simulink model "Fusion_Frame_Model_Architecture"  (R2018a)
settings: Solver=FixedStepAuto  StartTime=0.0  StopTime=SimulationTime  FixedStep=SamplingTime  RelTol=1e-3
undefined symbols (not defined in the file or in its folder): ACTIVATE_CAM, ACTIVATE_RAD, CAM1_detTimeStamp, CAM1_MeasNoise, CAM1_objClassID, CAM1_PX, CAM1_PY, CAM1_VX, CAM1_VY, CAM2_detTimeStamp, CAM2_MeasNoise, CAM2_objClassID, CAM2_PX, CAM2_PY, CAM2_VX, CAM2_VY, CAM3_detTimeStamp, CAM3_MeasNoise, CAM3_objClassID, CAM3_PX, CAM3_PY, CAM3_VX, CAM3_VY, CAM4_detTimeStamp, CAM4_MeasNoise, CAM4_objClassID, CAM4_PX, CAM4_PY, CAM4_VX, CAM4_VY, CAM5_detTimeStamp, CAM5_MeasNoise, CAM5_objClassID, CAM5_PX, CAM5_PY, CAM5_VX, CAM5_VY, CAM6_detTimeStamp, CAM6_MeasNoise, CAM6_objClassID, CAM6_PX, CAM6_PY, CAM6_VX, CAM6_VY, CAM7_detTimeStamp, CAM7_MeasNoise, CAM7_objClassID, CAM7_PX, CAM7_PY, CAM7_VX, CAM7_VY, CAM8_detTimeStamp, CAM8_MeasNoise, CAM8_objClassID, CAM8_PX, CAM8_PY, CAM8_VX, CAM8_VY, CAM_nMeas, CAM_TYPE ... (+181)
libraries: simulink_extras x4
(part 8 of 11)

== system Fusion_Frame_Model_Architecture/SENSOR_FUSION_SYSTEM/OBJECT_TRACKER_SENSOR_FUSION/SENSOR_LAYOUT_AND_CHRACTERIZATION/PRE_COMPUTE_SENSOR_FOV_GRID/CREATE_GRID/For Iterator Subsystem ==
  xIndex : Inport
  Cy : Inport  Port=2
  GridParam : Inport  Port=3
  CellIDArray : Inport  Port=4
  Compute_Grid_Cell_Cartesian_Coordinate : Subsystem
  Compute_Grid_Cell_Discreete_Index : Subsystem
  For Iterator : ForIterator  ResetStates=reset  IterationSource=external
  SET_DATA : Subsystem
  Terminator : Terminator
  Terminator1 : Terminator
  CellIDVectorUpd : Outport
  wires:
  Cy/1 -> For Iterator/1
  xIndex/1 -> Compute_Grid_Cell_Cartesian_Coordinate/2(x_Index)
  GridParam/1 -> Compute_Grid_Cell_Cartesian_Coordinate/1(GridParam), Compute_Grid_Cell_Discreete_Index/1(GridParam)
  Compute_Grid_Cell_Cartesian_Coordinate/2(y_Coordinate) -> Compute_Grid_Cell_Discreete_Index/3(y_coord)
  Compute_Grid_Cell_Cartesian_Coordinate/1(x_Coordinate) -> Compute_Grid_Cell_Discreete_Index/2(x_coord)
  For Iterator/1 -> Compute_Grid_Cell_Cartesian_Coordinate/3(y_Index)
  CellIDArray/1 -> SET_DATA/1(CellIDArray)
  SET_DATA/1(CellIDArrayUpd) -> CellIDVectorUpd/1
  Compute_Grid_Cell_Discreete_Index/1(CellID_x) -> Terminator/1
  Compute_Grid_Cell_Discreete_Index/2(CellID_y) -> Terminator1/1
  Compute_Grid_Cell_Discreete_Index/3(CellID) -> SET_DATA/2(CellID)

== system Fusion_Frame_Model_Architecture/SENSOR_FUSION_SYSTEM/OBJECT_TRACKER_SENSOR_FUSION/SENSOR_LAYOUT_AND_CHRACTERIZATION/SET_SENSOR_CALLIBRATION_PARAMETER/SET_CAMERA_SENSOR_PARAM/GET_DATA ==
  CAMSnsrParam : Inport
  Bus Selector : BusSelector  OutputSignals=CameraIntrinsics,CameraExtrinsics
  CameraIntrinsics : Outport
  CameraExtrinsics : Outport  Port=2
  wires:
  CAMSnsrParam/1 -> Bus Selector/1
  Bus Selector/2 -> CameraExtrinsics/1  "<CameraExtrinsics>"
  Bus Selector/1 -> CameraIntrinsics/1  "<CameraIntrinsics>"

== system Fusion_Frame_Model_Architecture/SENSOR_FUSION_SYSTEM/OBJECT_TRACKER_SENSOR_FUSION/SENSOR_LAYOUT_AND_CHRACTERIZATION/SET_SENSOR_CALLIBRATION_PARAMETER/SET_CAMERA_SENSOR_PARAM/SET_CAMERA_EXTRINSIC_PARAM ==
  CameraCalibParam : Inport
  INSTALLED_CAMERA_i : ForIterator  IterationLimit=nCameras
  SET_CAMERA_EXTRINSIC_PARAM : Subsystem
  CameraCalibParamSet : Outport
  wires:
  INSTALLED_CAMERA_i/1 -> SET_CAMERA_EXTRINSIC_PARAM/2(SensorID)
  SET_CAMERA_EXTRINSIC_PARAM/1(Out1) -> CameraCalibParamSet/1
  CameraCalibParam/1 -> SET_CAMERA_EXTRINSIC_PARAM/1(SensorParam)

== system Fusion_Frame_Model_Architecture/SENSOR_FUSION_SYSTEM/OBJECT_TRACKER_SENSOR_FUSION/SENSOR_LAYOUT_AND_CHRACTERIZATION/SET_SENSOR_CALLIBRATION_PARAMETER/SET_CAMERA_SENSOR_PARAM/SET_CAMERA_INTRINSIC_PARAM ==
  CameraCalibParam : Inport
  CAMERA_TYPE_i : ForIterator  IterationLimit=nCameraTypes
  SET_CAMERA_INTRINSIC_PARAM : Subsystem
  CameraCalibParamSet : Outport
  wires:
  CameraCalibParam/1 -> SET_CAMERA_INTRINSIC_PARAM/1(SensorParam)
  CAMERA_TYPE_i/1 -> SET_CAMERA_INTRINSIC_PARAM/2(SensorID)
  SET_CAMERA_INTRINSIC_PARAM/1(Out1) -> CameraCalibParamSet/1

== system Fusion_Frame_Model_Architecture/SENSOR_FUSION_SYSTEM/OBJECT_TRACKER_SENSOR_FUSION/SENSOR_LAYOUT_AND_CHRACTERIZATION/SET_SENSOR_CALLIBRATION_PARAMETER/SET_CAMERA_SENSOR_PARAM/SET_DATA ==
  CameraIntrinsics : Inport
  CameraExtrinsics : Inport  Port=2
  Bus Creator : BusCreator  Inputs=2  OutDataTypeStr=Bus: CAM_SENSOR_PARAM  NonVirtualBus=on
      settings: InheritFromInputs=off
  CAMSnsrParamUpd : Outport
  wires:
  Bus Creator/1 -> CAMSnsrParamUpd/1
  CameraIntrinsics/1 -> Bus Creator/1
  CameraExtrinsics/1 -> Bus Creator/2

== system Fusion_Frame_Model_Architecture/SENSOR_FUSION_SYSTEM/OBJECT_TRACKER_SENSOR_FUSION/SENSOR_LAYOUT_AND_CHRACTERIZATION/SET_SENSOR_CALLIBRATION_PARAMETER/SET_RADAR_SENSOR_PARAM/GET_DATA ==
  RADSnsrParam : Inport
  Bus Selector : BusSelector  OutputSignals=RadarIntrinsics,RadarExtrinsics
  <RadarIntrinsics> : Outport
  <RadarExtrinsics> : Outport  Port=2
  wires:
  Bus Selector/1 -> <RadarIntrinsics>/1  "<RadarIntrinsics>"
  RADSnsrParam/1 -> Bus Selector/1
  Bus Selector/2 -> <RadarExtrinsics>/1  "<RadarExtrinsics>"

== system Fusion_Frame_Model_Architecture/SENSOR_FUSION_SYSTEM/OBJECT_TRACKER_SENSOR_FUSION/SENSOR_LAYOUT_AND_CHRACTERIZATION/SET_SENSOR_CALLIBRATION_PARAMETER/SET_RADAR_SENSOR_PARAM/SET_DATA ==
  RadarIntrinsics : Inport
  RadarExtrinsics : Inport  Port=2
  Bus Creator : BusCreator  Inputs=2  OutDataTypeStr=Bus: RAD_SENSOR_PARAM  NonVirtualBus=on
      settings: InheritFromInputs=off
  RADSnsrParamUpd : Outport
  wires:
  RadarIntrinsics/1 -> Bus Creator/1  "RadarIntrnsics"
  RadarExtrinsics/1 -> Bus Creator/2  "RadarExtrinsics"
  Bus Creator/1 -> RADSnsrParamUpd/1

== system Fusion_Frame_Model_Architecture/SENSOR_FUSION_SYSTEM/OBJECT_TRACKER_SENSOR_FUSION/SENSOR_LAYOUT_AND_CHRACTERIZATION/SET_SENSOR_CALLIBRATION_PARAMETER/SET_RADAR_SENSOR_PARAM/SET_RADAR_EXTRINSIC_PARAM ==
  RadarCalibParam : Inport
  INSTALLED_RADAR_i : ForIterator  IterationLimit=nRadars
  SET_RADAR_EXTRINSIC_PARAM : Subsystem
  RadarCalibParamSet : Outport
  wires:
  RadarCalibParam/1 -> SET_RADAR_EXTRINSIC_PARAM/1(SensorParam)
  INSTALLED_RADAR_i/1 -> SET_RADAR_EXTRINSIC_PARAM/2(SensorID)
  SET_RADAR_EXTRINSIC_PARAM/1(RadarSensorParam) -> RadarCalibParamSet/1

== system Fusion_Frame_Model_Architecture/SENSOR_FUSION_SYSTEM/OBJECT_TRACKER_SENSOR_FUSION/SENSOR_LAYOUT_AND_CHRACTERIZATION/SET_SENSOR_CALLIBRATION_PARAMETER/SET_RADAR_SENSOR_PARAM/SET_RADAR_INTRINSIC_PARAM ==
  RadarCalibParam : Inport
  RADAR_TYPE_i : ForIterator  IterationLimit=nRadarTypes
  SET_RADAR_INTRINSIC_PARAM : Subsystem
  RadarCalibParamSet : Outport
  wires:
  RadarCalibParam/1 -> SET_RADAR_INTRINSIC_PARAM/1(SensorParam)
  RADAR_TYPE_i/1 -> SET_RADAR_INTRINSIC_PARAM/2(SensorID)
  SET_RADAR_INTRINSIC_PARAM/1(RadarIntrinsicParam) -> RadarCalibParamSet/1

== system Fusion_Frame_Model_Architecture/SENSOR_FUSION_SYSTEM/OBJECT_TRACKER_SENSOR_FUSION/SPATIAL_ALLIGNMENT1/CAMERA_MEASUREMENTS_SPATIAL_ALLIGNMENT/For Iterator Subsystem/For Iterator Subsystem ==
  CameraCalibration : Inport
  nMeas : Inport  Port=2
  CameraCAN : Inport  Port=3
  CoordinateTransformation1 : Subsystem  TreatAsAtomicUnit=on
  For Iterator : ForIterator  ResetStates=reset  IterationSource=external
  SetMeasurement1 : Subsystem
  Subsystem : Subsystem
  nValidMeas : Outport
  CameraMeasUpd : Outport  Port=2
  CameraMeasNoiseCovUpd : Outport  Port=3
  CameraMeasRefUpd : Outport  Port=4
  wires:
  nMeas/1 -> For Iterator/1
  CameraCalibration/1 -> CoordinateTransformation1/2(SensorParam)
  CameraCAN/1 -> Subsystem/1(measCAN)
  Subsystem/1(nValidMeasCnt) -> nValidMeas/1
  Subsystem/4(measID) -> SetMeasurement1/3(measID)
  Subsystem/2(isValid) -> CoordinateTransformation1/Action
  CoordinateTransformation1/1(measUpd) -> SetMeasurement1/1(measTransformed)
  For Iterator/1 -> SetMeasurement1/4(CamCANidx), Subsystem/2(measIdx)
  SetMeasurement1/1(CameraCTSMatUpd) -> CameraMeasUpd/1
  SetMeasurement1/2(CameraCTSNoiseCovMatUpd) -> CameraMeasNoiseCovUpd/1
  SetMeasurement1/3(CameraCTSRefUpd) -> CameraMeasRefUpd/1
  Subsystem/3(meas_i) -> CoordinateTransformation1/1(meas), SetMeasurement1/2(CameraMeasCAN)

== system Fusion_Frame_Model_Architecture/SENSOR_FUSION_SYSTEM/OBJECT_TRACKER_SENSOR_FUSION/SPATIAL_ALLIGNMENT1/CAMERA_MEASUREMENTS_SPATIAL_ALLIGNMENT/For Iterator Subsystem/InformationExtraction ==
  CameraCallibration : Inport
  CameraID : Inport  Port=2
  C1 : Inport  Port=3
  C2 : Inport  Port=4
  C3 : Inport  Port=5
  C4 : Inport  Port=6
  C5 : Inport  Port=7
  C6 : Inport  Port=8
  C7 : Inport  Port=9
  C8 : Inport  Port=10
  StartingIndexes : Inport  Port=11
  Bus Selector : BusSelector  OutputSignals=nMeas
  Multiport Switch : MultiPortSwitch  Inputs=8
  Reshape : Reshape  OutputDimensionality=Row vector (2-D)
  Selector : Selector  NumberOfDimensions=2  InputPortWidth=3  IndexOptions=Select all,Index vector (port)  Indices=[1 3],1  OutputSizes=1,1
  Selector1 : Selector  NumberOfDimensions=2  InputPortWidth=3  IndexOptions=Select all,Index vector (port)  Indices=[1 3],1  OutputSizes=1,1
  CameraCalib : Outport
  nCameraMeas : Outport  Port=2
  CameraCANBus : Outport  Port=3
  MeasStartingIdx : Outport  Port=4
  wires:
  CameraCallibration/1 -> Selector/1
  Selector/1 -> CameraCalib/1, Bus Selector/1
  Bus Selector/1 -> nCameraMeas/1  "<nMeas>"
  CameraID/1 -> Selector1/2, Multiport Switch/1, Selector/2
  C1/1 -> Multiport Switch/2
  C2/1 -> Multiport Switch/3
  C3/1 -> Multiport Switch/4
  C4/1 -> Multiport Switch/5
  C5/1 -> Multiport Switch/6
  C6/1 -> Multiport Switch/7
  Multiport Switch/1 -> Reshape/1
  Selector1/1 -> MeasStartingIdx/1
  StartingIndexes/1 -> Selector1/1
  Reshape/1 -> CameraCANBus/1
  C7/1 -> Multiport Switch/8
  C8/1 -> Multiport Switch/9

== system Fusion_Frame_Model_Architecture/SENSOR_FUSION_SYSTEM/OBJECT_TRACKER_SENSOR_FUSION/SPATIAL_ALLIGNMENT1/CAMERA_MEASUREMENTS_SPATIAL_ALLIGNMENT/For Iterator Subsystem/Subsystem ==
  SnsrIndex : Inport
  nValidMeas : Inport  Port=2
  CameraCTSMeas : Inport  Port=3
  CameraCTSNoiseCOV : Inport  Port=4
  CameraCTSRef : Inport  Port=5
  StartIdx : Inport  Port=6
  Add : Sum
  Assignment : Assignment  NumberOfDimensions=2  DiagnosticForDimensions=Warning  IndexOptions=Assign all,Index vector (port)  Indices=1,1  OutputSizes=1,1
  Assignment1 : Assignment  NumberOfDimensions=2  DiagnosticForDimensions=Warning  IndexOptions=Assign all,Starting index (port)  Indices=1,1  OutputSizes=1,1
  Assignment2 : Assignment  NumberOfDimensions=3  DiagnosticForDimensions=Warning  IndexOptions=Assign all,Assign all,Starting index (port)  Indices=1,1,1  OutputSizes=1,1,1
  Assignment3 : Assignment  NumberOfDimensions=2  DiagnosticForDimensions=Warning  IndexOptions=Assign all,Starting index (port)  Indices=1,1  OutputSizes=1,1
  Constant2 : Constant  Value=int32(1)
  Data Type Conversion : DataTypeConversion  OutDataTypeStr=uint16
  Reshape : Reshape  OutputDimensionality=Row vector (2-D)
  Unit Delay : UnitDelay  InitialCondition=single(zeros(2, 1600))  SampleTime=-1
  Unit Delay1 : UnitDelay  InitialCondition=uint16(zeros(1,8))  SampleTime=-1
  Unit Delay2 : UnitDelay  InitialCondition=single(zeros(2, 2, 1600))  SampleTime=-1
  Unit Delay3 : UnitDelay  InitialCondition=uint16(zeros(2, 1600))  SampleTime=-1
  nValidMeasVector : Outport
  CTSMat : Outport  Port=2
  CTSMatNoiseCOV : Outport  Port=3
  CTSMatRef : Outport  Port=4
  wires:
  nValidMeas/1 -> Data Type Conversion/1
  SnsrIndex/1 -> Assignment/3
  Assignment/1 -> [nValidMeas], nValidMeasVector/1
  Unit Delay1/1 -> Reshape/1
  CameraCTSMeas/1 -> Assignment1/2
  Assignment1/1 -> [CTSMat], CTSMat/1
  StartIdx/1 -> Add/1
  Constant2/1 -> Add/2
  Data Type Conversion/1 -> Assignment/2
  Reshape/1 -> Assignment/1
  Unit Delay/1 -> Assignment1/1
  Unit Delay2/1 -> Assignment2/1
  CameraCTSNoiseCOV/1 -> Assignment2/2
  Add/1 -> Assignment3/3, Assignment2/3, Assignment1/3
  Assignment2/1 -> [CTSMatCov], CTSMatNoiseCOV/1
  Assignment3/1 -> [CTSRefMat], CTSMatRef/1
  CameraCTSRef/1 -> Assignment3/2
  Unit Delay3/1 -> Assignment3/1
  [nValidMeas] -> Unit Delay1/1
  [CTSMat] -> Unit Delay/1
  [CTSMatCov] -> Unit Delay2/1
  [CTSRefMat] -> Unit Delay3/1

== system Fusion_Frame_Model_Architecture/SENSOR_FUSION_SYSTEM/OBJECT_TRACKER_SENSOR_FUSION/SPATIAL_ALLIGNMENT1/CAMERA_MEASUREMENTS_SPATIAL_ALLIGNMENT/RadarMeasurementIndexes2/FIND1 ==
  measIdx : Inport
  Add : Sum
  Assignment : Assignment  NumberOfDimensions=2  DiagnosticForDimensions=Warning  IndexOptions=Assign all,Index vector (port)  Indices=1,1  OutputSizes=1,1
  Constant : Constant  Value=uint16(0)
  Constant1 : Constant  Value=uint16(1)
  Constant2 : Constant  Value=uint16(0)
  Constant3 : Constant  Value=int32(1)
  For Iterator : ForIterator  ResetStates=reset  IterationLimit=maxNumMeasCamera
  NotEqual : RelationalOperator  Operator=~=  OutDataTypeStr=boolean  RndMeth=Simplest
  NotEqual1 : RelationalOperator  Operator=~=  OutDataTypeStr=boolean  RndMeth=Simplest
  Reshape : Reshape  OutputDimensionality=Row vector (2-D)
  Selector : Selector  NumberOfDimensions=2  InputPortWidth=3  IndexOptions=Select all,Index vector (port)  Indices=[1 3],1  OutputSizes=1,1
  Switch : Switch  Criteria=u2 ~= 0
  Switch1 : Switch  Criteria=u2 ~= 0
  Switch2 : Switch  Criteria=u2 ~= 0
  Unit Delay : UnitDelay  InitialCondition=uint16(0)  SampleTime=-1
  Unit Delay1 : UnitDelay  InitialCondition=int32(1)  SampleTime=-1
  Unit Delay2 : UnitDelay  InitialCondition=int32(ones(1,maxNumMeasCamera))  SampleTime=-1
  ValidIndex : Outport
  wires:
  Constant/1 -> NotEqual/2, Switch/3
  Add/1 -> [idx], Unit Delay/1
  Selector/1 -> NotEqual/1
  measIdx/1 -> Selector/1
  Unit Delay2/1 -> Reshape/1
  Unit Delay/1 -> Add/2
  Unit Delay1/1 -> Switch1/3
  Assignment/1 -> ValidIndex/1, Unit Delay2/1
  Reshape/1 -> Assignment/1
  [idx] -> Switch2/1, NotEqual1/1
  Constant2/1 -> NotEqual1/2
  [isValid] -> Switch1/2
  NotEqual/1 -> Switch/2, [isValid]
  For Iterator/1 -> [measIdx], Selector/2
  Constant1/1 -> Switch/1
  Constant3/1 -> Switch2/3
  Switch2/1 -> Assignment/3
  Switch/1 -> Add/1
  NotEqual1/1 -> Switch2/2
  Switch1/1 -> Unit Delay1/1, Assignment/2
  [measIdx] -> Switch1/1

== system Fusion_Frame_Model_Architecture/SENSOR_FUSION_SYSTEM/OBJECT_TRACKER_SENSOR_FUSION/SPATIAL_ALLIGNMENT1/CAMERA_MEASUREMENTS_SPATIAL_ALLIGNMENT/StartingIndexes1/CallibrationInfoExtractor ==
  SnsrCallib : Inport
  Bus Selector{,1..7} (8 alike) : BusSelector  OutputSignals=nMeas
  Selector : Selector  InputPortWidth=nCameras  IndexOptions=Index vector (dialog)  Indices=1  OutputSizes=1
  Selector1 : Selector  InputPortWidth=nCameras  IndexOptions=Index vector (dialog)  Indices=2  OutputSizes=1
  Selector2 : Selector  InputPortWidth=nCameras  IndexOptions=Index vector (dialog)  Indices=3  OutputSizes=1
  Selector3 : Selector  InputPortWidth=nCameras  IndexOptions=Index vector (dialog)  Indices=4  OutputSizes=1
  Selector4 : Selector  InputPortWidth=nCameras  IndexOptions=Index vector (dialog)  Indices=5  OutputSizes=1
  Selector5 : Selector  InputPortWidth=nCameras  IndexOptions=Index vector (dialog)  Indices=7  OutputSizes=1
  Selector6 : Selector  InputPortWidth=nCameras  IndexOptions=Index vector (dialog)  Indices=6  OutputSizes=1
  Selector7 : Selector  InputPortWidth=nCameras  IndexOptions=Index vector (dialog)  Indices=8  OutputSizes=1
  Terminator : Terminator
  C1nMeas : Outport
  C2nMeas : Outport  Port=2
  C3nMeas : Outport  Port=3
  C4nMeas : Outport  Port=4
  C5nMeas : Outport  Port=5
  C6nMeas : Outport  Port=6
  C7nMeas : Outport  Port=7
  wires:
  Bus Selector4/1 -> C5nMeas/1  "<nMeas>"
  Selector4/1 -> Bus Selector4/1
  Bus Selector1/1 -> C2nMeas/1  "<nMeas>"
  Selector1/1 -> Bus Selector1/1
  Selector2/1 -> Bus Selector2/1
  Bus Selector2/1 -> C3nMeas/1  "<nMeas>"
  Selector6/1 -> Bus Selector5/1
  Selector/1 -> Bus Selector/1
  Selector3/1 -> Bus Selector3/1
  Bus Selector3/1 -> C4nMeas/1  "<nMeas>"
  Bus Selector/1 -> C1nMeas/1  "<nMeas>"
  Bus Selector5/1 -> C6nMeas/1  "<nMeas>"
  Selector5/1 -> Bus Selector6/1
  Bus Selector6/1 -> C7nMeas/1  "<nMeas>"
  Bus Selector7/1 -> Terminator/1  "<nMeas>"
  Selector7/1 -> Bus Selector7/1
  SnsrCallib/1 -> Selector7/1, Selector5/1, Selector6/1, Selector4/1, Selector3/1, Selector2/1, Selector1/1, Selector/1

== system Fusion_Frame_Model_Architecture/SENSOR_FUSION_SYSTEM/OBJECT_TRACKER_SENSOR_FUSION/SPATIAL_ALLIGNMENT1/CAMERA_MEASUREMENTS_SPATIAL_ALLIGNMENT/StartingIndexes1/Subsystem ==
  C1nMeas : Inport
  C2nMeas : Inport  Port=2
  C3nMeas : Inport  Port=3
  C4nMeas : Inport  Port=4
  C5nMeas : Inport  Port=5
  C6nMeas : Inport  Port=6
  C7nMeas : Inport  Port=7
  Add{,1..5} (6 alike) : Sum
  Constant : Constant  Value=int32(0)
  Data Type Conversion{,1..6} (7 alike) : DataTypeConversion  OutDataTypeStr=int32
  Mux : Mux  Inputs=8
  Reshape : Reshape  OutputDimensionality=Row vector (2-D)
  StartingIndexes : Outport
  wires:
  [C1] -> Mux/1
  Add/1 -> [C3], Add1/1
  Add1/1 -> [C4], Add2/1
  Data Type Conversion3/1 -> Add2/2
  [C4] -> Mux/4
  [C2] -> Mux/2
  Add3/1 -> Add4/1, [C6]
  Constant/1 -> [C1]
  Add2/1 -> [C5], Add3/1
  [C5] -> Mux/5
  [C6] -> Mux/6
  C5nMeas/1 -> Data Type Conversion4/1
  Data Type Conversion/1 -> [C2], Add/1
  [C3] -> Mux/3
  Data Type Conversion1/1 -> Add/2
  Data Type Conversion2/1 -> Add1/2
  Data Type Conversion4/1 -> Add3/2
  C3nMeas/1 -> Data Type Conversion2/1
  C1nMeas/1 -> Data Type Conversion/1
  C2nMeas/1 -> Data Type Conversion1/1
  Mux/1 -> Reshape/1
  C4nMeas/1 -> Data Type Conversion3/1
  Reshape/1 -> StartingIndexes/1
  C6nMeas/1 -> Data Type Conversion5/1
  C7nMeas/1 -> Data Type Conversion6/1
  Data Type Conversion5/1 -> Add4/2
  Data Type Conversion6/1 -> Add5/2
  Add4/1 -> [C7], Add5/1
  Add5/1 -> [C8]
  [C7] -> Mux/7
  [C8] -> Mux/8

== system Fusion_Frame_Model_Architecture/SENSOR_FUSION_SYSTEM/OBJECT_TRACKER_SENSOR_FUSION/SPATIAL_ALLIGNMENT1/RADAR_MEASUREMENTS_SPATIAL_ALLIGNMENT/RADAR_MEASUREMENTS_SPATIAL_ALLIGNMENT/COORDINATE_TRANSFORMATION ==
  RadarCalibration : Inport
  nMeas : Inport  Port=2
  RadarCAN : Inport  Port=3
  COORDINATE_TRANSFORMATION : Subsystem  TreatAsAtomicUnit=on
  GET_DATA : Subsystem
  MEASUREMENT_LOOP : ForIterator  ResetStates=reset  IterationSource=external
  SET_DATA : Subsystem
  nValidMeas : Outport
  RadarMeasUpd : Outport  Port=2
  RadarMeasNoiseCovUpd : Outport  Port=3
  RadarMeasRefUpd : Outport  Port=4
  wires:
  nMeas/1 -> MEASUREMENT_LOOP/1
  RadarCalibration/1 -> COORDINATE_TRANSFORMATION/2(SensorParam)
  RadarCAN/1 -> GET_DATA/1(measCAN)
  MEASUREMENT_LOOP/1 -> GET_DATA/2(measIdx), SET_DATA/4(RadCANidx)
  GET_DATA/3(meas_i) -> SET_DATA/2(RadarMeasCAN), COORDINATE_TRANSFORMATION/1(meas)
  GET_DATA/2(nValidMeasCnt) -> nValidMeas/1
  GET_DATA/4(measID) -> SET_DATA/3(measID)
  COORDINATE_TRANSFORMATION/1(measUpd) -> SET_DATA/1(measTransformed)
  SET_DATA/1(RadarCTSMatUpd) -> RadarMeasUpd/1
  GET_DATA/1(isValid) -> COORDINATE_TRANSFORMATION/Action
  SET_DATA/3(RadarCTSRefUpd) -> RadarMeasRefUpd/1
  SET_DATA/2(RadarCTSNoiseCovMatUpd) -> RadarMeasNoiseCovUpd/1

== system Fusion_Frame_Model_Architecture/SENSOR_FUSION_SYSTEM/OBJECT_TRACKER_SENSOR_FUSION/SPATIAL_ALLIGNMENT1/RADAR_MEASUREMENTS_SPATIAL_ALLIGNMENT/RADAR_MEASUREMENTS_SPATIAL_ALLIGNMENT/GET_DATA ==
  RadarCallibration : Inport
  RadarID : Inport  Port=2
  R1 : Inport  Port=3
  R2 : Inport  Port=4
  R3 : Inport  Port=5
  R4 : Inport  Port=6
  R5 : Inport  Port=7
  R6 : Inport  Port=8
  StartingIndexes : Inport  Port=9
  Bus Selector : BusSelector  OutputSignals=nMeas
  Multiport Switch : MultiPortSwitch  Inputs=6
  Reshape : Reshape  OutputDimensionality=Row vector (2-D)
  Selector : Selector  NumberOfDimensions=2  InputPortWidth=3  IndexOptions=Select all,Index vector (port)  Indices=[1 3],1  OutputSizes=1,1
  Selector1 : Selector  NumberOfDimensions=2  InputPortWidth=3  IndexOptions=Select all,Index vector (port)  Indices=[1 3],1  OutputSizes=1,1
  RadarCalib : Outport
  nRadarMeas : Outport  Port=2
  RadarCANBus : Outport  Port=3
  MeasStartingIdx : Outport  Port=4
  wires:
  RadarCallibration/1 -> Selector/1
  Selector/1 -> RadarCalib/1, Bus Selector/1
  Bus Selector/1 -> nRadarMeas/1  "<nMeas>"
  RadarID/1 -> Selector1/2, Selector/2, Multiport Switch/1
  R1/1 -> Multiport Switch/2
  R2/1 -> Multiport Switch/3
  R3/1 -> Multiport Switch/4
  R4/1 -> Multiport Switch/5
  R5/1 -> Multiport Switch/6
  R6/1 -> Multiport Switch/7
  Multiport Switch/1 -> Reshape/1
  Selector1/1 -> MeasStartingIdx/1
  StartingIndexes/1 -> Selector1/1
  Reshape/1 -> RadarCANBus/1

== system Fusion_Frame_Model_Architecture/SENSOR_FUSION_SYSTEM/OBJECT_TRACKER_SENSOR_FUSION/SPATIAL_ALLIGNMENT1/RADAR_MEASUREMENTS_SPATIAL_ALLIGNMENT/RADAR_MEASUREMENTS_SPATIAL_ALLIGNMENT/SET_DATA ==
  SnsrIndex : Inport
  nValidMeas : Inport  Port=2
  RadarCTSMeas : Inport  Port=3
  RadarCTSNoiseCOV : Inport  Port=4
  RadarCTSRef : Inport  Port=5
  StartIdx : Inport  Port=6
  Add : Sum
  Assignment : Assignment  NumberOfDimensions=2  DiagnosticForDimensions=Warning  IndexOptions=Assign all,Index vector (port)  Indices=1,1  OutputSizes=1,1
  Assignment1 : Assignment  NumberOfDimensions=2  DiagnosticForDimensions=Warning  IndexOptions=Assign all,Starting index (port)  Indices=1,1  OutputSizes=1,1
  Assignment2 : Assignment  NumberOfDimensions=3  DiagnosticForDimensions=Warning  IndexOptions=Assign all,Assign all,Starting index (port)  Indices=1,1,1  OutputSizes=1,1,1
  Assignment3 : Assignment  NumberOfDimensions=2  DiagnosticForDimensions=Warning  IndexOptions=Assign all,Starting index (port)  Indices=1,1  OutputSizes=1,1
  Constant2 : Constant  Value=int32(1)
  Data Type Conversion : DataTypeConversion  OutDataTypeStr=uint16
  Reshape : Reshape  OutputDimensionality=Row vector (2-D)
  Unit Delay : UnitDelay  InitialCondition=single(zeros(2, 1200))  SampleTime=-1
  Unit Delay1 : UnitDelay  InitialCondition=uint16(zeros(1,6))  SampleTime=-1
  Unit Delay2 : UnitDelay  InitialCondition=single(zeros(2, 2, 1200))  SampleTime=-1
  Unit Delay3 : UnitDelay  InitialCondition=uint16(zeros(2, 1200))  SampleTime=-1
  nValidMeasVector : Outport
  CTSMat : Outport  Port=2
  CTSMatNoiseCOV : Outport  Port=3
  CTSMatRef : Outport  Port=4
  wires:
  nValidMeas/1 -> Data Type Conversion/1
  SnsrIndex/1 -> Assignment/3
  Assignment/1 -> [nValidMeas], nValidMeasVector/1
  Unit Delay1/1 -> Reshape/1
  RadarCTSMeas/1 -> Assignment1/2
  Assignment1/1 -> [CTSMat], CTSMat/1
  StartIdx/1 -> Add/1
  Constant2/1 -> Add/2
  Data Type Conversion/1 -> Assignment/2
  Reshape/1 -> Assignment/1
  Unit Delay/1 -> Assignment1/1
  Unit Delay2/1 -> Assignment2/1
  RadarCTSNoiseCOV/1 -> Assignment2/2
  Add/1 -> Assignment3/3, Assignment2/3, Assignment1/3
  Assignment2/1 -> [CTSMatCov], CTSMatNoiseCOV/1
  Assignment3/1 -> [CTSRefMat], CTSMatRef/1
  RadarCTSRef/1 -> Assignment3/2
  Unit Delay3/1 -> Assignment3/1
  [nValidMeas] -> Unit Delay1/1
  [CTSMat] -> Unit Delay/1
  [CTSMatCov] -> Unit Delay2/1
  [CTSRefMat] -> Unit Delay3/1

== system Fusion_Frame_Model_Architecture/SENSOR_FUSION_SYSTEM/OBJECT_TRACKER_SENSOR_FUSION/SPATIAL_ALLIGNMENT1/RADAR_MEASUREMENTS_SPATIAL_ALLIGNMENT/SET_MEASUREMENTS/FIND ==
  measIdx : Inport
  Add : Sum
  Assignment : Assignment  NumberOfDimensions=2  DiagnosticForDimensions=Warning  IndexOptions=Assign all,Index vector (port)  Indices=1,1  OutputSizes=1,1
  Constant : Constant  Value=uint16(0)
  Constant1 : Constant  Value=uint16(1)
  Constant2 : Constant  Value=uint16(0)
  Constant3 : Constant  Value=int32(1)
  For Iterator : ForIterator  ResetStates=reset  IterationLimit=maxNumMeasRadar
  NotEqual : RelationalOperator  Operator=~=  OutDataTypeStr=boolean  RndMeth=Simplest
  NotEqual1 : RelationalOperator  Operator=~=  OutDataTypeStr=boolean  RndMeth=Simplest
  Reshape : Reshape  OutputDimensionality=Row vector (2-D)
  Selector : Selector  NumberOfDimensions=2  InputPortWidth=3  IndexOptions=Select all,Index vector (port)  Indices=[1 3],1  OutputSizes=1,1
  Switch : Switch  Criteria=u2 ~= 0
  Switch1 : Switch  Criteria=u2 ~= 0
  Switch2 : Switch  Criteria=u2 ~= 0
  Unit Delay : UnitDelay  InitialCondition=uint16(0)  SampleTime=-1
  Unit Delay1 : UnitDelay  InitialCondition=int32(1)  SampleTime=-1
  Unit Delay2 : UnitDelay  InitialCondition=int32(ones(1,maxNumMeasRadar))  SampleTime=-1
  ValidIndex : Outport
  wires:
  Constant/1 -> NotEqual/2, Switch/3
  Add/1 -> [idx], Unit Delay/1
  Selector/1 -> NotEqual/1
  measIdx/1 -> Selector/1
  Unit Delay2/1 -> Reshape/1
  Unit Delay/1 -> Add/2
  Unit Delay1/1 -> Switch1/3
  Assignment/1 -> ValidIndex/1, Unit Delay2/1
  Reshape/1 -> Assignment/1
  [idx] -> Switch2/1, NotEqual1/1
  Constant2/1 -> NotEqual1/2
  [isValid] -> Switch1/2
  NotEqual/1 -> Switch/2, [isValid]
  For Iterator/1 -> [measIdx], Selector/2
  Constant1/1 -> Switch/1
  Constant3/1 -> Switch2/3
  Switch2/1 -> Assignment/3
  Switch/1 -> Add/1
  NotEqual1/1 -> Switch2/2
  Switch1/1 -> Unit Delay1/1, Assignment/2
  [measIdx] -> Switch1/1

== system Fusion_Frame_Model_Architecture/SENSOR_FUSION_SYSTEM/OBJECT_TRACKER_SENSOR_FUSION/SPATIAL_ALLIGNMENT1/RADAR_MEASUREMENTS_SPATIAL_ALLIGNMENT/StartingIndexes1/CallibrationInfoExtractor ==
  SnsrCallib : Inport
  Bus Selector{,1..5} (6 alike) : BusSelector  OutputSignals=nMeas
  Selector : Selector  InputPortWidth=nRadars  IndexOptions=Index vector (dialog)  Indices=1  OutputSizes=1
  Selector1 : Selector  InputPortWidth=nRadars  IndexOptions=Index vector (dialog)  Indices=2  OutputSizes=1
  Selector2 : Selector  InputPortWidth=nRadars  IndexOptions=Index vector (dialog)  Indices=3  OutputSizes=1
  Selector3 : Selector  InputPortWidth=nRadars  IndexOptions=Index vector (dialog)  Indices=4  OutputSizes=1
  Selector4 : Selector  InputPortWidth=nRadars  IndexOptions=Index vector (dialog)  Indices=5  OutputSizes=1
  Selector5 : Selector  InputPortWidth=nRadars  IndexOptions=Index vector (dialog)  Indices=6  OutputSizes=1
  Terminator : Terminator
  R1nMeas : Outport
  R2nMeas : Outport  Port=2
  R3nMeas : Outport  Port=3
  R4nMeas : Outport  Port=4
  R5nMeas : Outport  Port=5
  wires:
  Bus Selector4/1 -> R5nMeas/1  "<nMeas>"
  Selector4/1 -> Bus Selector4/1
  SnsrCallib/1 -> Selector1/1, Selector2/1, Selector3/1, Selector5/1, Selector4/1, Selector/1
  Bus Selector1/1 -> R2nMeas/1  "<nMeas>"
  Selector1/1 -> Bus Selector1/1
  Selector2/1 -> Bus Selector2/1
  Bus Selector2/1 -> R3nMeas/1  "<nMeas>"
  Selector5/1 -> Bus Selector5/1
  Selector/1 -> Bus Selector/1
  Selector3/1 -> Bus Selector3/1
  Bus Selector5/1 -> Terminator/1  "<nMeas>"
  Bus Selector3/1 -> R4nMeas/1  "<nMeas>"
  Bus Selector/1 -> R1nMeas/1  "<nMeas>"

== system Fusion_Frame_Model_Architecture/SENSOR_FUSION_SYSTEM/OBJECT_TRACKER_SENSOR_FUSION/SPATIAL_ALLIGNMENT1/RADAR_MEASUREMENTS_SPATIAL_ALLIGNMENT/StartingIndexes1/Subsystem ==
  R1nMeas : Inport
  R2nMeas : Inport  Port=2
  R3nMeas : Inport  Port=3
  R4nMeas : Inport  Port=4
  R5nMeas : Inport  Port=5
  Add{,1..3} (4 alike) : Sum
  Constant : Constant  Value=int32(0)
  Data Type Conversion{,1..4} (5 alike) : DataTypeConversion  OutDataTypeStr=int32
  Mux : Mux  Inputs=6
  Reshape : Reshape  OutputDimensionality=Row vector (2-D)
  StartingIndexes : Outport
  wires:
  [R1] -> Mux/1
  Add/1 -> [R3], Add1/1
  Add1/1 -> [R4], Add2/1
  Data Type Conversion3/1 -> Add2/2
  [R4] -> Mux/4
  [R2] -> Mux/2
  Add3/1 -> [R6]
  Constant/1 -> [R1]
  Add2/1 -> [R5], Add3/1
  [R5] -> Mux/5
  [R6] -> Mux/6
  R5nMeas/1 -> Data Type Conversion4/1
  Data Type Conversion/1 -> [R2], Add/1
  [R3] -> Mux/3
  Data Type Conversion1/1 -> Add/2
  Data Type Conversion2/1 -> Add1/2
  Data Type Conversion4/1 -> Add3/2
  R3nMeas/1 -> Data Type Conversion2/1
  R1nMeas/1 -> Data Type Conversion/1
  R2nMeas/1 -> Data Type Conversion1/1
  Mux/1 -> Reshape/1
  R4nMeas/1 -> Data Type Conversion3/1
  Reshape/1 -> StartingIndexes/1

== system Fusion_Frame_Model_Architecture/SENSOR_FUSION_SYSTEM/OBJECT_TRACKER_SENSOR_FUSION/CAMERA_HOMOGENEOUS_FUSION/NEAREST_NEIGHBOUR_CLUSTERING_FOR_CAMERA_MEASUREMENT/NN_MEASUREMENT_GROUPING_WITHIN_EPS/COMPUTE_MEAN_IF_CLUSTER_FORMED/COMPUTE_COVARIANCE ==
  covariance_sum : Inport
  n : Inport  Port=2
  Constant : Constant  Value=uint16(1)
  Constant1 : Constant  Value=uint16(0)
  Constant2 : Constant  Value=single(eye(2))
  Divide : Product  Inputs=*/
  Subtract : Sum  Inputs=-+
  Switch : Switch  Criteria=u2 > Threshold  Threshold=uint16(1)
  Switch1 : Switch  Criteria=u2 > Threshold  Threshold=uint16(1)
  Covariance : Outport
  wires:
  n/1 -> [nPts], Switch/2
  Constant/1 -> Switch/1
  covariance_sum/1 -> Divide/1
  Constant1/1 -> Switch/3
  Switch/1 -> Subtract/1
  [nPts] -> Subtract/2
  Subtract/1 -> Divide/2
  [nPts] -> Switch1/2
  Divide/1 -> Switch1/1
  Switch1/1 -> Covariance/1
  Constant2/1 -> Switch1/3

== system Fusion_Frame_Model_Architecture/SENSOR_FUSION_SYSTEM/OBJECT_TRACKER_SENSOR_FUSION/CAMERA_HOMOGENEOUS_FUSION/NEAREST_NEIGHBOUR_CLUSTERING_FOR_CAMERA_MEASUREMENT/NN_MEASUREMENT_GROUPING_WITHIN_EPS/COMPUTE_MEAN_IF_CLUSTER_FORMED/COMPUTE_COVARIANCE_SUM ==
  mean : Inport
  MeasArray : Inport  Port=2
  nPoints : Inport  Port=3
  ClusterMembers : Inport  Port=4
  Add1 : Sum
  Bus Selector : BusSelector  OutputSignals=MeasArray
  For Iterator : ForIterator  ResetStates=reset  IterationSource=external
  Matrix Multiply : Product  Multiplication=Matrix(*)
  Selector : Selector  NumberOfDimensions=2  InputPortWidth=3  IndexOptions=Select all,Index vector (port)  Indices=[1 3],1  OutputSizes=1,1
  Selector1 : Selector  NumberOfDimensions=2  InputPortWidth=3  IndexOptions=Select all,Index vector (port)  Indices=[1 3],1  OutputSizes=1,1
  Subtract : Sum  Inputs=+-
  Transpose : Math  Operator=transpose  SaturateOnIntegerOverflow=on
  Unit Delay : UnitDelay  InitialCondition=single(zeros(2,2))  SampleTime=-1
  ClusterCovSUM : Outport
  wires:
  nPoints/1 -> For Iterator/1
  ClusterMembers/1 -> Selector/1
  For Iterator/1 -> Selector/2
  MeasArray/1 -> Bus Selector/1
  Bus Selector/1 -> Selector1/1  "<MeasArray>"
  Selector/1 -> Selector1/2
  Unit Delay/1 -> Add1/1
  Add1/1 -> Unit Delay/1, ClusterCovSUM/1
  Subtract/1 -> Matrix Multiply/1, Transpose/1
  Transpose/1 -> Matrix Multiply/2
  Matrix Multiply/1 -> Add1/2
  Selector1/1 -> Subtract/2
  mean/1 -> Subtract/1

== system Fusion_Frame_Model_Architecture/SENSOR_FUSION_SYSTEM/OBJECT_TRACKER_SENSOR_FUSION/CAMERA_HOMOGENEOUS_FUSION/NEAREST_NEIGHBOUR_CLUSTERING_FOR_CAMERA_MEASUREMENT/NN_MEASUREMENT_GROUPING_WITHIN_EPS/COMPUTE_MEAN_IF_CLUSTER_FORMED/COMPUTE_MEAN ==
  mean_sum : Inport
  n : Inport  Port=2
  Divide : Product  Inputs=*/
  mean : Outport
  wires:
  mean_sum/1 -> Divide/1
  Divide/1 -> mean/1
  n/1 -> Divide/2

== system Fusion_Frame_Model_Architecture/SENSOR_FUSION_SYSTEM/OBJECT_TRACKER_SENSOR_FUSION/CAMERA_HOMOGENEOUS_FUSION/NEAREST_NEIGHBOUR_CLUSTERING_FOR_CAMERA_MEASUREMENT/NN_MEASUREMENT_GROUPING_WITHIN_EPS/COMPUTE_MEAN_IF_CLUSTER_FORMED/COMPUTE_MEAN_SUM ==
  ClusterMembers : Inport
  nPoints : Inport  Port=2
  MeasArray : Inport  Port=3
  Add1 : Sum
  Bus Selector : BusSelector  OutputSignals=MeasArray
  For Iterator : ForIterator  ResetStates=reset  IterationSource=external
  Selector : Selector  NumberOfDimensions=2  InputPortWidth=3  IndexOptions=Select all,Index vector (port)  Indices=[1 3],1  OutputSizes=1,1
  Selector1 : Selector  NumberOfDimensions=2  InputPortWidth=3  IndexOptions=Select all,Index vector (port)  Indices=[1 3],1  OutputSizes=1,1
  Unit Delay : UnitDelay  InitialCondition=single(0)  SampleTime=-1
  ClusterMeanSUM : Outport
  wires:
  nPoints/1 -> For Iterator/1
  ClusterMembers/1 -> Selector/1
  For Iterator/1 -> Selector/2
  MeasArray/1 -> Bus Selector/1
  Bus Selector/1 -> Selector1/1  "<MeasArray>"
  Selector/1 -> Selector1/2
  Selector1/1 -> Add1/2
  Unit Delay/1 -> Add1/1
  Add1/1 -> ClusterMeanSUM/1, Unit Delay/1

== system Fusion_Frame_Model_Architecture/SENSOR_FUSION_SYSTEM/OBJECT_TRACKER_SENSOR_FUSION/CAMERA_HOMOGENEOUS_FUSION/NEAREST_NEIGHBOUR_CLUSTERING_FOR_CAMERA_MEASUREMENT/NN_MEASUREMENT_GROUPING_WITHIN_EPS/COMPUTE_MEAN_IF_CLUSTER_FORMED/GET_DATA ==
  CLSTR : Inport
  Bus Selector : BusSelector  OutputSignals=ClusterSizes,nClusters,ClusterMember
  Selector : Selector  NumberOfDimensions=2  InputPortWidth=3  IndexOptions=Select all,Index vector (port)  Indices=[1 3],1  OutputSizes=1,1
  nPts : Outport
  <ClusterMember> : Outport  Port=2
  wires:
  Bus Selector/1 -> Selector/1  "<ClusterSizes>"
  Selector/1 -> nPts/1
  Bus Selector/2 -> Selector/2  "<nClusters>"
  Bus Selector/3 -> <ClusterMember>/1  "<ClusterMember>"
  CLSTR/1 -> Bus Selector/1

== system Fusion_Frame_Model_Architecture/SENSOR_FUSION_SYSTEM/OBJECT_TRACKER_SENSOR_FUSION/CAMERA_HOMOGENEOUS_FUSION/NEAREST_NEIGHBOUR_CLUSTERING_FOR_CAMERA_MEASUREMENT/NN_MEASUREMENT_GROUPING_WITHIN_EPS/For Iterator Subsystem/If Action Subsystem ==
  CLSTR_DATA : Inport
  Action Port : ActionPort  ActionType=else
  Constant : Constant  Value=uint16(0)
  CLSTR_DATA_NO_UPD : Outport
  nPtsEpsNoUpd : Outport  Port=2
  wires:
  CLSTR_DATA/1 -> CLSTR_DATA_NO_UPD/1
  Constant/1 -> nPtsEpsNoUpd/1

== system Fusion_Frame_Model_Architecture/SENSOR_FUSION_SYSTEM/OBJECT_TRACKER_SENSOR_FUSION/CAMERA_HOMOGENEOUS_FUSION/NEAREST_NEIGHBOUR_CLUSTERING_FOR_CAMERA_MEASUREMENT/NN_MEASUREMENT_GROUPING_WITHIN_EPS/For Iterator Subsystem/MERGE_SIGNALS ==
  CLSTR_NO_UPD : Inport
  nPtsEpsNoUpd : Inport  Port=2
  nPtsUpd : Inport  Port=3
  CLSTR_UPD : Inport  Port=4
  Merge : Merge
  Merge1 : Merge
  nPtsEps : Outport
  CLSTR_DATA : Outport  Port=2
  wires:
  CLSTR_NO_UPD/1 -> Merge1/1
  Merge1/1 -> CLSTR_DATA/1
  nPtsEpsNoUpd/1 -> Merge/1
  Merge/1 -> nPtsEps/1
  nPtsUpd/1 -> Merge/2
  CLSTR_UPD/1 -> Merge1/2

== system Fusion_Frame_Model_Architecture/SENSOR_FUSION_SYSTEM/OBJECT_TRACKER_SENSOR_FUSION/CAMERA_HOMOGENEOUS_FUSION/NEAREST_NEIGHBOUR_CLUSTERING_FOR_CAMERA_MEASUREMENT/NN_MEASUREMENT_GROUPING_WITHIN_EPS/For Iterator Subsystem/NN ==
  CLSTR_DATA : Inport  OutDataTypeStr=Bus: CLUSTER_DATA_STRUCT_SNSR
  measArray : Inport  Port=2
  idx_i : Inport  Port=3
  Action Port : ActionPort  ActionType=then
  PERFORM_NN_CLUSTERING : Subsystem
  SET_CLUSTER_ID_AND_UPDATE_NUMBER_OF_CLUSTERS : Subsystem
  Subsystem : Subsystem
  nPtsEps : Outport
  CLSTR_DATA_UPD : Outport  Port=2  OutDataTypeStr=Bus: CLUSTER_DATA_STRUCT_SNSR
  wires:
  idx_i/1 -> PERFORM_NN_CLUSTERING/4(idx_i)
  SET_CLUSTER_ID_AND_UPDATE_NUMBER_OF_CLUSTERS/2(CLUSTER_DATA) -> PERFORM_NN_CLUSTERING/3(CLSTR_DATA)
  SET_CLUSTER_ID_AND_UPDATE_NUMBER_OF_CLUSTERS/1(nRadMeas) -> PERFORM_NN_CLUSTERING/1(nMeas)
  CLSTR_DATA/1 -> SET_CLUSTER_ID_AND_UPDATE_NUMBER_OF_CLUSTERS/1(CLUSTERING_DATA)
  measArray/1 -> SET_CLUSTER_ID_AND_UPDATE_NUMBER_OF_CLUSTERS/2(CAM_MEAS_CTS), [meas]
  [meas] -> PERFORM_NN_CLUSTERING/2(measArray)
  Subsystem/1(ClstrSize) -> nPtsEps/1
  PERFORM_NN_CLUSTERING/1(CLSTR_DATA_UPD) -> Subsystem/1(CLSTR_DATA), CLSTR_DATA_UPD/1

== system Fusion_Frame_Model_Architecture/SENSOR_FUSION_SYSTEM/OBJECT_TRACKER_SENSOR_FUSION/CAMERA_HOMOGENEOUS_FUSION/NEAREST_NEIGHBOUR_CLUSTERING_FOR_CAMERA_MEASUREMENT/NN_MEASUREMENT_GROUPING_WITHIN_EPS/For Iterator Subsystem/Subsystem ==
  idx_i : Inport
  CLSTR_in : Inport  Port=2
  Bus Selector : BusSelector  OutputSignals=isMeasVisitedFlag
  Logical Operator1 : Logic  Operator=NOT  AllPortsSameDT=off  OutDataTypeStr=boolean
  Selector1 : Selector  NumberOfDimensions=2  InputPortWidth=3  IndexOptions=Select all,Index vector (port)  Indices=1,1  OutputSizes=1,1
  Unit Delay : UnitDelay  InitialCondition=CLSTR_SNSR_DELAY_INIT  SampleTime=-1
  isNotVisited : Outport
  CLSTR_out : Outport  Port=2
  wires:
  Logical Operator1/1 -> isNotVisited/1
  Selector1/1 -> Logical Operator1/1
  idx_i/1 -> Selector1/2
  CLSTR_in/1 -> Unit Delay/1
  Bus Selector/1 -> Selector1/1  "<isMeasVisitedFlag>"
  Unit Delay/1 -> CLSTR_out/1, Bus Selector/1

== system Fusion_Frame_Model_Architecture/SENSOR_FUSION_SYSTEM/OBJECT_TRACKER_SENSOR_FUSION/CAMERA_HOMOGENEOUS_FUSION/NEAREST_NEIGHBOUR_CLUSTERING_FOR_CAMERA_MEASUREMENT/NN_MEASUREMENT_GROUPING_WITHIN_EPS/Subsystem3/GET_DATA_FROM_BUS ==
  CLSTR_DATA : Inport
  Bus Selector : BusSelector  OutputSignals=ClusterCenter,ClusterCovariance,nClusters
  <ClusterCenter> : Outport
  <ClusterCovariance> : Outport  Port=2
  <nClusters> : Outport  Port=3
  wires:
  Bus Selector/3 -> <nClusters>/1  "<nClusters>"
  Bus Selector/1 -> <ClusterCenter>/1  "<ClusterCenter>"
  CLSTR_DATA/1 -> Bus Selector/1
  Bus Selector/2 -> <ClusterCovariance>/1  "<ClusterCovariance>"

== system Fusion_Frame_Model_Architecture/SENSOR_FUSION_SYSTEM/OBJECT_TRACKER_SENSOR_FUSION/CAMERA_HOMOGENEOUS_FUSION/NEAREST_NEIGHBOUR_CLUSTERING_FOR_CAMERA_MEASUREMENT/NN_MEASUREMENT_GROUPING_WITHIN_EPS/Subsystem3/SET_DATA_TO_BUS ==
  CLSTR_DATA : Inport
  Mean_ARRAY : Inport  Port=2
  Cov_ARRAY : Inport  Port=3
  Bus Creator : BusCreator  Inputs=7  OutDataTypeStr=Bus: CLUSTER_DATA_STRUCT_SNSR  NonVirtualBus=on
      settings: InheritFromInputs=off
  Bus Selector1 : BusSelector  OutputSignals=ClusterCenter,ClusterCovariance,ClusterSizes,ClusterToMeasAssignment,isMeasVisitedFlag,nClusters,ClusterMember
  Constant1 : Constant  Value=ClusterMemArray_SNSR
  Reshape1 : Reshape  OutputDimensionality=Row vector (2-D)
  Terminator1 : Terminator
  Terminator2 : Terminator
  Terminator3 : Terminator
  "CLSTR_DATA_UPD " : Outport
  wires:
  Constant1/1 -> Reshape1/1  "ClusterMember"
  Bus Selector1/5 -> Bus Creator/5  "<isMeasVisitedFlag>"
  Cov_ARRAY/1 -> Bus Creator/2  "ClusterCovariance"
  Mean_ARRAY/1 -> Bus Creator/1  "ClusterCenter"
  Bus Selector1/1 -> Terminator2/1  "<ClusterCenter>"
  Bus Selector1/7 -> Terminator1/1  "<ClusterMember>"
  Bus Selector1/2 -> Terminator3/1  "<ClusterCovariance>"
  Bus Selector1/3 -> Bus Creator/3  "<ClusterSizes>"
  Reshape1/1 -> Bus Creator/7  "ClusterMember"
  Bus Selector1/4 -> Bus Creator/4  "<ClusterToMeasAssignment>"
  Bus Selector1/6 -> Bus Creator/6  "<nClusters>"
  Bus Creator/1 -> "CLSTR_DATA_UPD "/1
  CLSTR_DATA/1 -> Bus Selector1/1

== system Fusion_Frame_Model_Architecture/SENSOR_FUSION_SYSTEM/OBJECT_TRACKER_SENSOR_FUSION/CAMERA_HOMOGENEOUS_FUSION/NEAREST_NEIGHBOUR_CLUSTERING_FOR_CAMERA_MEASUREMENT/NN_MEASUREMENT_GROUPING_WITHIN_EPS/Subsystem3/UPDATE_CLUSTER_DATA ==
  Center_ARRAY : Inport
  Cov_ARRAY : Inport  Port=2
  ID : Inport  Port=3
  mean1 : Inport  Port=4
  mean2 : Inport  Port=5
  Cov1 : Inport  Port=6
  Cov2 : Inport  Port=7
  FLAG : Inport  Port=8
  Assignment : Assignment  NumberOfDimensions=2  DiagnosticForDimensions=Warning  IndexOptions=Assign all,Index vector (port)  Indices=1,1  OutputSizes=1,1
  Assignment1 : Assignment  NumberOfDimensions=3  DiagnosticForDimensions=Warning  IndexOptions=Assign all,Assign all,Index vector (port)  Indices=1,1,1  OutputSizes=1,1,1
  Merge : Merge
  Merge2 : Merge
  Selector : Selector  NumberOfDimensions=2  InputPortWidth=3  IndexOptions=Select all,Index vector (port)  Indices=[1 3],1  OutputSizes=1,1
  Selector1 : Selector  NumberOfDimensions=3  InputPortWidth=3  IndexOptions=Select all,Select all,Index vector (port)  Indices=[1 3],1,1  OutputSizes=1,1,1
  Switch : Switch  Criteria=u2 ~= 0
  Switch1 : Switch  Criteria=u2 ~= 0
  CenterUpd : Outport
  CovUpd : Outport  Port=2
  wires:
  Selector/1 -> Switch/3
  Merge2/1 -> Switch1/1
  Cov_ARRAY/1 -> Assignment1/1, Selector1/1
  mean1/1 -> Merge/1
  Selector1/1 -> Switch1/3
  Merge/1 -> Switch/1
  Switch1/1 -> Assignment1/2
  Switch/1 -> Assignment/2
  Cov2/1 -> Merge2/2
  Assignment1/1 -> CovUpd/1
  Assignment/1 -> CenterUpd/1
  Cov1/1 -> Merge2/1
  mean2/1 -> Merge/2
  FLAG/1 -> [FLAG]
  [FLAG] -> Switch/2
  [FLAG] -> Switch1/2
  [ID] -> Assignment/3, Selector/2
  ID/1 -> [ID], Assignment1/3, Selector1/2
  Center_ARRAY/1 -> Selector/1, Assignment/1

== system Fusion_Frame_Model_Architecture/SENSOR_FUSION_SYSTEM/OBJECT_TRACKER_SENSOR_FUSION/RADAR_HOMOGENEOUS_FUSION/GATING/MEASUREMENT_TO_TRACK_GATING_AND_LOGLIKELIHOOD_COMPUTATION/GATE_MEASUREMENTS_AND_COMPUTE_LIKELIHOOD/GATE_MEASUREMENT_AND_COMPUTE_LOG_LIKELIHOOD ==
  mDist : Inport
  GatedMeasFlagIn : Inport  Port=2
  TrackIdx : Inport  Port=3
  innovCov : Inport  Port=4
  LogLikelihoodArrayIn : Inport  Port=5
  P_D : Inport  Port=6
  measIdx : Inport  Port=7
  Assignment : Assignment  NumberOfDimensions=2  DiagnosticForDimensions=Warning  IndexOptions=Index vector (port),Index vector (port)  Indices=1,1  OutputSizes=1,1
  Assignment1 : Assignment  NumberOfDimensions=2  DiagnosticForDimensions=Warning  IndexOptions=Index vector (port),Index vector (port)  Indices=1,1  OutputSizes=1,1
  Constant : Constant  Value=GammaSq
  Constant1 : Constant  Value=true
  Constant2 : Constant  Value=false
  Constant3 : Constant  Value=INVALID_LIKELIHOOD
  Constant4 : Constant  Value=pi
  Constant5 : Constant  Value=single(0.5)
  Constant6 : Constant  Value=single(0.5)
  Gain : Gain  Gain=2
  GreaterThan : RelationalOperator  Operator=<=  OutDataTypeStr=boolean  RndMeth=Simplest
  Log : Math  Operator=log  SaturateOnIntegerOverflow=on
  MATLAB Function1 : MATLAB Function  TreatAsAtomicUnit=on
  Multiply : Product
  Multiply1 : Product
  Multiply2 : Product
  Square : Math  Operator=square  SaturateOnIntegerOverflow=on
  Subtract : Sum  Inputs=--
  Switch : Switch  Criteria=u2 ~= 0
  Switch1 : Switch  Criteria=u2 ~= 0
  Switch2 : Switch  Criteria=u2 > Threshold  Threshold=int32(1)
  Switch3 : Switch  Criteria=u2 > Threshold  Threshold=int32(1)
  Terminator4 : Terminator
  Unit Delay : UnitDelay  SampleTime=-1
  Unit Delay1 : UnitDelay  SampleTime=-1
  GatedMeasFlagArray : Outport
  LogLikelihoodArray : Outport  Port=2
  wires:
  innovCov/1 -> MATLAB Function1/1(InnoCov)
  P_D/1 -> Terminator4/1
  Constant/1 -> GreaterThan/2
  GreaterThan/1 -> [isGated], Switch/2
  Constant1/1 -> Switch/1
  Constant2/1 -> Switch/3
  Constant3/1 -> Switch1/3
  [isGated] -> Switch1/2
  Constant4/1 -> Gain/1
  Gain/1 -> Square/1
  Square/1 -> Multiply/1
  MATLAB Function1/1(detInnoCov) -> Multiply/2
  Multiply/1 -> Log/1
  Log/1 -> Multiply1/1
  Constant5/1 -> Multiply1/2
  Multiply1/1 -> Subtract/2
  Subtract/1 -> Switch1/1
  Multiply2/1 -> Subtract/1
  mDist/1 -> Multiply2/1, GreaterThan/1
  Constant6/1 -> Multiply2/2
  Switch/1 -> Assignment/2
  Switch1/1 -> Assignment1/2
  Assignment/1 -> GatedMeasFlagArray/1, Unit Delay/1
  measIdx/1 -> [measIdx], Assignment/4
  TrackIdx/1 -> [objIdx], Assignment/3
  [objIdx] -> Assignment1/3
  [measIdx] -> Assignment1/4
  GatedMeasFlagIn/1 -> Switch2/3
  Unit Delay/1 -> Switch2/1
  [measIdx] -> Switch2/2
  LogLikelihoodArrayIn/1 -> Switch3/3
  [measIdx] -> Switch3/2
  Unit Delay1/1 -> Switch3/1
  Assignment1/1 -> Unit Delay1/1, LogLikelihoodArray/1
  Switch2/1 -> Assignment/1
  Switch3/1 -> Assignment1/1

== system Fusion_Frame_Model_Architecture/SENSOR_FUSION_SYSTEM/OBJECT_TRACKER_SENSOR_FUSION/RADAR_HOMOGENEOUS_FUSION/GATING/MEASUREMENT_TO_TRACK_GATING_AND_LOGLIKELIHOOD_COMPUTATION/GATE_MEASUREMENTS_AND_COMPUTE_LIKELIHOOD/GET_DATA ==
  MEAS : Inport
  SNSR_PARAM : Inport  Port=2
  measIdx : Inport  Port=3
  Bus Selector : BusSelector  OutputSignals=MeasArray,MeasCovariance,MeasRef
  Bus Selector1 : BusSelector  OutputSignals=RadarIntrinsics,RadarExtrinsics
  Bus Selector2 : BusSelector  OutputSignals=ProbOfDetection
  Bus Selector3 : BusSelector  OutputSignals=RadarType
  Selector : Selector  NumberOfDimensions=2  InputPortWidth=3  IndexOptions=Select all,Index vector (port)  Indices=[1 3],1  OutputSizes=1,1
  Selector1 : Selector  NumberOfDimensions=3  InputPortWidth=3  IndexOptions=Select all,Select all,Index vector (port)  Indices=[1 3],1,1  OutputSizes=1,1,1
  Selector2 : Selector  NumberOfDimensions=2  InputPortWidth=3  IndexOptions=Select all,Index vector (port)  Indices=[1 3],1  OutputSizes=1,1
  Selector3 : Selector  NumberOfDimensions=2  InputPortWidth=3  IndexOptions=Select all,Index vector (port)  Indices=[1 3],1  OutputSizes=1,1
  Selector4 : Selector  NumberOfDimensions=2  InputPortWidth=3  IndexOptions=Index vector (dialog),Index vector (port)  Indices=2,1  OutputSizes=1,1
  measVector : Outport
  measCov : Outport  Port=2
  P_D : Outport  Port=3
  wires:
  Bus Selector/2 -> Selector1/1  "<MeasCovariance>"
  Selector/1 -> measVector/1
  Selector1/1 -> measCov/1
  Bus Selector/1 -> Selector/1  "<MeasArray>"
  SNSR_PARAM/1 -> Bus Selector1/1
  MEAS/1 -> Bus Selector/1
  Bus Selector1/2 -> Selector2/1  "<RadarExtrinsics>"
  [snsrId] -> Selector2/2
  Selector2/1 -> Bus Selector3/1
  Bus Selector1/1 -> Selector3/1  "<RadarIntrinsics>"
  Bus Selector3/1 -> Selector3/2  "<RadarType>"
  Selector3/1 -> Bus Selector2/1
  Bus Selector2/1 -> P_D/1  "<ProbOfDetection>"
  Bus Selector/3 -> Selector4/1  "<MeasRef>"
  Selector4/1 -> [snsrId]
  measIdx/1 -> Selector/2, Selector1/2, Selector4/2

== system Fusion_Frame_Model_Architecture/SENSOR_FUSION_SYSTEM/OBJECT_TRACKER_SENSOR_FUSION/RADAR_HOMOGENEOUS_FUSION/GATING/MEASUREMENT_TO_TRACK_GATING_AND_LOGLIKELIHOOD_COMPUTATION/GATE_MEASUREMENTS_AND_COMPUTE_LIKELIHOOD/MAHALANOBIS_DISTANCE ==
  meas : Inport
  measCov : Inport  Port=2
  TrackStateVector : Inport  Port=3
  TrackErrCov : Inport  Port=4
  Constant1 : Constant  Value=MeasModelCA2PxPy
  MATLAB Function : MATLAB Function  TreatAsAtomicUnit=on
  Matrix Multiply : Product  Multiplication=Matrix(*)
  Matrix Multiply1 : Product  Inputs=3  Multiplication=Matrix(*)
  Matrix Multiply2 : Product  Inputs=3  Multiplication=Matrix(*)
  Subtract : Sum  Inputs=+-
  Subtract1 : Sum
  Transpose : Math  Operator=transpose  SaturateOnIntegerOverflow=on
  Transpose1 : Math  Operator=transpose  SaturateOnIntegerOverflow=on
  mDist : Outport
  innovCov : Outport  Port=2
  wires:
  Matrix Multiply/1 -> Subtract/2
  Transpose/1 -> Matrix Multiply1/3
  meas/1 -> Subtract/1
  Transpose1/1 -> Matrix Multiply2/1
  TrackErrCov/1 -> Matrix Multiply1/2
  Subtract/1 -> Transpose1/1, [innov]
  [innov] -> Matrix Multiply2/3
  Constant1/1 -> Transpose/1, Matrix Multiply1/1, Matrix Multiply/1
  TrackStateVector/1 -> Matrix Multiply/2
  Matrix Multiply1/1 -> Subtract1/1
  measCov/1 -> Subtract1/2
  Matrix Multiply2/1 -> mDist/1
  Subtract1/1 -> innovCov/1, MATLAB Function/1(InnoCov)
  MATLAB Function/1(InnoCovInverse) -> Matrix Multiply2/2

== system Fusion_Frame_Model_Architecture/SENSOR_FUSION_SYSTEM/OBJECT_TRACKER_SENSOR_FUSION/RADAR_HOMOGENEOUS_FUSION/SIMPLYFIED_DBSCAN_FOR_RADAR_MEASUREMENT_GROUPING/DBSCAN_MEASUREMENT_GROUPING/COMPUTE_MEAN_IF_CLUSTER_FORMED/COMPUTE_COVARIANCE ==
  covariance_sum : Inport
  n : Inport  Port=2
  Constant : Constant  Value=uint16(1)
  Constant1 : Constant  Value=uint16(0)
  Constant2 : Constant  Value=single(eye(2))
  Divide : Product  Inputs=*/
  Subtract : Sum  Inputs=-+
  Switch : Switch  Criteria=u2 > Threshold  Threshold=uint16(1)
  Switch1 : Switch  Criteria=u2 > Threshold  Threshold=uint16(1)
  Covariance : Outport
  wires:
  n/1 -> [nPts], Switch/2
  Constant/1 -> Switch/1
  covariance_sum/1 -> Divide/1
  Constant1/1 -> Switch/3
  Switch/1 -> Subtract/1
  [nPts] -> Subtract/2
  Subtract/1 -> Divide/2
  [nPts] -> Switch1/2
  Divide/1 -> Switch1/1
  Switch1/1 -> Covariance/1
  Constant2/1 -> Switch1/3

== system Fusion_Frame_Model_Architecture/SENSOR_FUSION_SYSTEM/OBJECT_TRACKER_SENSOR_FUSION/RADAR_HOMOGENEOUS_FUSION/SIMPLYFIED_DBSCAN_FOR_RADAR_MEASUREMENT_GROUPING/DBSCAN_MEASUREMENT_GROUPING/COMPUTE_MEAN_IF_CLUSTER_FORMED/COMPUTE_COVARIANCE_SUM ==
  mean : Inport
  MeasArray : Inport  Port=2
  nPoints : Inport  Port=3
  ClusterMembers : Inport  Port=4
  Add1 : Sum
  Bus Selector : BusSelector  OutputSignals=MeasArray
  For Iterator : ForIterator  ResetStates=reset  IterationSource=external
  Matrix Multiply : Product  Multiplication=Matrix(*)
  Selector : Selector  NumberOfDimensions=2  InputPortWidth=3  IndexOptions=Select all,Index vector (port)  Indices=[1 3],1  OutputSizes=1,1
  Selector1 : Selector  NumberOfDimensions=2  InputPortWidth=3  IndexOptions=Select all,Index vector (port)  Indices=[1 3],1  OutputSizes=1,1
  Subtract : Sum  Inputs=+-
  Transpose : Math  Operator=transpose  SaturateOnIntegerOverflow=on
  Unit Delay : UnitDelay  InitialCondition=single(zeros(2,2))  SampleTime=-1
  ClusterCovSUM : Outport
  wires:
  nPoints/1 -> For Iterator/1
  ClusterMembers/1 -> Selector/1
  For Iterator/1 -> Selector/2
  MeasArray/1 -> Bus Selector/1
  Bus Selector/1 -> Selector1/1  "<MeasArray>"
  Selector/1 -> Selector1/2
  Unit Delay/1 -> Add1/1
  Add1/1 -> Unit Delay/1, ClusterCovSUM/1
  Subtract/1 -> Matrix Multiply/1, Transpose/1
  Transpose/1 -> Matrix Multiply/2
  Matrix Multiply/1 -> Add1/2
  Selector1/1 -> Subtract/2
  mean/1 -> Subtract/1

== system Fusion_Frame_Model_Architecture/SENSOR_FUSION_SYSTEM/OBJECT_TRACKER_SENSOR_FUSION/RADAR_HOMOGENEOUS_FUSION/SIMPLYFIED_DBSCAN_FOR_RADAR_MEASUREMENT_GROUPING/DBSCAN_MEASUREMENT_GROUPING/COMPUTE_MEAN_IF_CLUSTER_FORMED/COMPUTE_MEAN ==
  mean_sum : Inport
  n : Inport  Port=2
  Divide : Product  Inputs=*/
  mean : Outport
  wires:
  mean_sum/1 -> Divide/1
  Divide/1 -> mean/1
  n/1 -> Divide/2
